simulink library "KL_DeviceData_HvsAct"  (Simulink 7.8)
settings: Solver=ode45  StartTime=0.0  StopTime=10.0  RelTol=1e-3
settings Model: Creator=KLJS168  LastModifiedBy=KLJS168

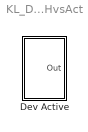
== system KL_DeviceData_HvsAct ==
  Dev Active : Subsystem

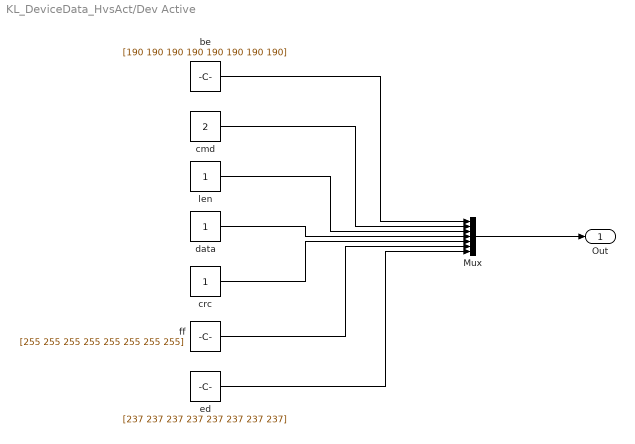
== system KL_DeviceData_HvsAct/Dev Active ==
  Mux : Mux  Inputs=7
  be : Constant  Value=[190 190 190 190 190 190 190 190]
  cmd : Constant  Value=2
  crc : Constant
  data : Constant
  ed : Constant  Value=[237 237 237 237 237 237 237 237]
  ff : Constant  Value=[255 255 255 255 255 255 255 255]
  len : Constant
  Out : Outport
  wires:
  Mux/1 -> Out/1
  ed/1 -> Mux/7
  ff/1 -> Mux/6
  crc/1 -> Mux/5
  data/1 -> Mux/4
  len/1 -> Mux/3
  cmd/1 -> Mux/2
  be/1 -> Mux/1
